simulink model "uz_ParameterID6ph"  (R2021b)
settings: Solver=FixedStepDiscrete  StartTime=0.0  StopTime=160  FixedStep=0.000005  RelTol=1e-3  EnableMultiTasking=on
model workspace (MATLAB code in the model file):
  | cmdLim = Simulink.Parameter;
  | cmdLim.Value = 15;
  | cmdLim.Description = 'Limit for controlling the maximum surface command angle.';
  | cmdLim.Min = 0;
  | cmdLim.Max = 90;
  | cmdLim.DocUnits = 'deg';
  | 
  | dispGain = Simulink.Parameter;
  | dispGain.Value = 0.75;
  | dispGain.Description = 'Gain applied to the displacement error.';
  | dispGain.Min = 0;
  | dispGain.Max = [];
  | dispGain.DocUnits = 'deg/sec/deg';
  | 
  | dispLim = Simulink.Parameter;
  | dispLim.Value = 30;
  | dispLim.Description = 'Limit for controlling the maximum commanded angle.';
  | dispLim.Min = 0;
  | dispLim.Max = 180;
  | dispLim.DocUnits = 'deg';
  | 
  | intGain = Simulink.Parameter;
  | intGain.Value = 0.5;
  | intGain.Description = 'Gain applied to the integral error.';
  | intGain.Min = 0;
  | intGain.Max = [];
  | intGain.DocUnits = 'deg/sec/deg/sec';
  | 
  | intLim = Simulink.Parameter;
  | intLim.Value = 5;
  | intLim.Description = 'Limit for controlling the maximum commanded angle.';
  | intLim.Min = 0;
  | intLim.Max = 90;
  | intLim.DocUnits = 'deg';
  | 
  | rateGain = Simulink.Parameter;
  | rateGain.Value = 2;
  | rateGain.Description = 'Gain applied to the rate error.';
  | rateGain.Min = 0;
  | rateGain.Max = [];
  | rateGain.DocUnits = 'deg/deg/sec';
  | 
  | rateLim = Simulink.Parameter;
  | rateLim.Value = 6;
  | rateLim.Description = 'Limit for controlling the maximum commanded angle.';
  | rateLim.Min = 0;
  | rateLim.Max = 180;
  | rateLim.DocUnits = 'deg/sec';
  | 
  | hdgGain = Simulink.Parameter;
  | hdgGain.Value = 0.015;
values from neighbouring files (symbols this model uses):
  c = 2/6*cat(1,tl1,tl2,tl3,tl4,tl5,tl6)    [Parameter_Init_Buehler_201_6ph.m]
  d_d_TMS = 0.005    [Parameter_Init_Buehler_201.m]
  d_f_hardware = 200000    [Parameter_Init_Buehler_201.m]
  d_f_states = 20000    [Parameter_Init_Buehler_201.m]
  d_i_max = 15    [Parameter_Init_Buehler_201.m]
  d_i_min = -d_i_max    (= -15)    [Parameter_Init_Buehler_201.m]
  d_I_n = 8    [Parameter_Init_Buehler_201.m]
  d_J_Coupling_M_E = 2e-6    (= 2e-06)    [Parameter_Init_Buehler_201.m]
  d_J_Coupling_M_Ms = 2e-20    [Parameter_Init_Buehler_201.m]
  d_J_Ms_L = d_J_Ms_M    (= 1.26363648e-05)    [Parameter_Init_Buehler_201.m]
  d_J_Ms_M = 0.5*0.5*((0.5*d_d_Ms)^4)*3.14*d_l_Ms*d_rho_Ms    (= 1.26363648e-05)    [Parameter_Init_Buehler_201.m]
  d_Ki_id = 162.47    [Parameter_Init_Buehler_201.m]
  d_Ki_iq = 162.47    [Parameter_Init_Buehler_201.m]
  d_Ki_n = 1.982    [Parameter_Init_Buehler_201.m]
  d_Kp_id = 0.369    [Parameter_Init_Buehler_201.m]
  d_Kp_iq = 0.369    [Parameter_Init_Buehler_201.m]
  d_Kp_n = 0.198    [Parameter_Init_Buehler_201.m]
  d_L_d = 0.00031    [Parameter_Init_Buehler_201.m]
  d_L_q = 0.00033    [Parameter_Init_Buehler_201.m]
  d_n_n = 3200    [Parameter_Init_Buehler_201.m]
  d_p = 4    [Parameter_Init_Buehler_201.m]
  d_psi_pm = 0.0075    [Parameter_Init_Buehler_201.m]
  d_R_ph = d_R_ph_ph/2    (= 0.089)    [Parameter_Init_Buehler_201.m]
  d_y_max = 10    [Parameter_Init_Buehler_201.m]
  d_y_min = -d_y_max    (= -10)    [Parameter_Init_Buehler_201.m]
  V_DC = 24    [Parameter_Init_Buehler_201.m]
undefined symbols (not defined in the file or in its folder): i_dq, i_dq_ref, n_ref, ts_ps, V_abc, v_dq
libraries: fl_lib x66, nesl_utility x51, ee_lib x38, simulink x14, spsTriangleGeneratorLib x3, spsabctodq0Lib x2, spsAlphaBetaZerotodq0Lib x2, spsdq0toabcLib x1
(part 5 of 6)

== system uz_ParameterID6ph/Hardware/coupling m. shaft/Inertia ==
  Trägheitsmoment3 : fl_lib/Mechanical/Rotational Elements/Inertia  Commented=on  inertia=d_J_Coupling_M_Ms kg*m^2  num_ports=foundation.enum.numPorts2.one  w_specify=off  w_priority=High  w=0 rad/s  w_nominal_specify=off  w_nominal_unit=rad/s  w_nominal_value=1  t_specify=off  t_priority=None  t=0 N*m  t_nominal_specify=off  t_nominal_unit=N*m  t_nominal_value=1
      settings: AttributesFormatString=J in [%<inertia_unit>]
  Input : PMIOPort  Side=Left
  output : PMIOPort  Port=2  Side=Right
  connections:
  Input/RConn1 -- Trägheitsmoment3/LConn1 -- output/RConn1

== system uz_ParameterID6ph/Hardware/coupling m. shaft/Spring Damper System ==
  Rotational Spring : fl_lib/Mechanical/Rotational Elements/Rotational Spring  spr_rate=d_c_Coupling_M_Ms N*m/rad  w_specify=off  w_priority=None  w=0 rad/s  w_nominal_specify=off  w_nominal_unit=rad/s  w_nominal_value=1  t_specify=off  t_priority=None  t=0 N*m  t_nominal_specify=off  t_nominal_unit=N*m  t_nominal_value=1  phi_specify=off  phi_priority=High  phi=0 rad  phi_nominal_specify=off  phi_nominal_unit=rad  phi_nominal_value=1
  Trägheitsmoment1 : fl_lib/Mechanical/Rotational Elements/Inertia  inertia=d_J_Coupling_M_Ms/2 kg*m^2  num_ports=foundation.enum.numPorts2.one  w_specify=off  w_priority=High  w=0 rad/s  w_nominal_specify=off  w_nominal_unit=rad/s  w_nominal_value=1  t_specify=off  t_priority=None  t=0 N*m  t_nominal_specify=off  t_nominal_unit=N*m  t_nominal_value=1
      settings: AttributesFormatString=J in [%<inertia_unit>]
  Trägheitsmoment3 : fl_lib/Mechanical/Rotational Elements/Inertia  inertia=d_J_Coupling_M_Ms/2 kg*m^2  num_ports=foundation.enum.numPorts2.one  w_specify=off  w_priority=High  w=0 rad/s  w_nominal_specify=off  w_nominal_unit=rad/s  w_nominal_value=1  t_specify=off  t_priority=None  t=0 N*m  t_nominal_specify=off  t_nominal_unit=N*m  t_nominal_value=1
      settings: AttributesFormatString=J in [%<inertia_unit>]
  dm : fl_lib/Mechanical/Rotational Elements/Rotational Damper  Commented=on  D=0 N*m/(rad/s)  w_specify=off  w_priority=None  w=0 rad/s  w_nominal_specify=off  w_nominal_unit=rad/s  w_nominal_value=1  t_specify=off  t_priority=None  t=0 N*m  t_nominal_specify=off  t_nominal_unit=N*m  t_nominal_value=1
  Input : PMIOPort  Side=Left
  output : PMIOPort  Port=2  Side=Right
  connections:
  Rotational Spring/LConn1 -- dm/LConn1 -- Input/RConn1 -- Trägheitsmoment3/LConn1
  Trägheitsmoment1/LConn1 -- Rotational Spring/RConn1 -- dm/RConn1 -- output/RConn1

== system uz_ParameterID6ph/Hardware1/maschine_models/Connected_VSD ==
  Mechanical Rotational Reference2 : fl_lib/Mechanical/Rotational Elements/Mechanical Rotational Reference
  Open Circuit : fl_lib/Electrical/Electrical Elements/Open Circuit  v_specify=off  v_priority=None  v=0 V  v_nominal_specify=off  v_nominal_unit=V  v_nominal_value=1
      settings: SourceProductBaseCode=SS
  Phase Splitter3 : ee_lib/Connectors & References/Phase Splitter
      settings: SourceProductBaseCode=PS
  Phase Splitter4 : ee_lib/Connectors & References/Phase Splitter
      settings: SourceProductBaseCode=PS
  Simscape Component1 : SimscapeComponentBlock  SourceFile=PMSM_6ph_VSD_Rockhill_singleN  ComponentPath=PMSM_6ph_VSD_Rockhill_singleN  ComponentVariants="[\"PMSM_6ph_VSD_Rockhill_singleN\"]"  ComponentVariantNames="[\"PMSM_6ph_VSD_Rockhill_singleN\"]"  ClassName=PMSM_6ph_VSD_Rockhill_singleN  SchemaVersion=1  psi_pm=1 Wb  L_d=1 H  L_q=1 H  L_ls=0.00016 H  Rs=1 Ohm  p=1  n=9  i_a1_specify=off  i_a1_priority=None  i_a1=0 A  i_a1_nominal_specify=off  i_a1_nominal_unit=A  i_a1_nominal_value=1  i_b1_specify=off  i_b1_priority=None  i_b1=0 A  i_b1_nominal_specify=off  i_b1_nominal_unit=A  i_b1_nominal_value=1  i_c1_specify=off  i_c1_priority=None  i_c1=0 A  i_c1_nominal_specify=off  i_c1_nominal_unit=A  i_c1_nominal_value=1  i_a2_specify=off  i_a2_priority=None  i_a2=0 A  i_a2_nominal_specify=off  i_a2_nominal_unit=A  i_a2_nominal_value=1  i_b2_specify=off  i_b2_priority=None  i_b2=0 A  i_b2_nominal_specify=off  i_b2_nominal_unit=A  i_b2_nominal_value=1  i_c2_specify=off  i_c2_priority=None  i_c2=0 A  i_c2_nominal_specify=off  i_c2_nominal_unit=A  i_c2_nominal_value=1  i_d_specify=off  i_d_priority=None  i_d=0 A  i_d_nominal_specify=off  i_d_nominal_unit=A  i_d_nominal_value=1  i_q_specify=off  i_q_priority=None  i_q=0 A  i_q_nominal_specify=off  i_q_nominal_unit=A  i_q_nominal_value=1  i_a_specify=off  i_a_priority=None  i_a=0 A  i_a_nominal_specify=off  i_a_nominal_unit=A  i_a_nominal_value=1  i_b_specify=off  i_b_priority=None  i_b=0 A  i_b_nominal_specify=off  i_b_nominal_unit=A  i_b_nominal_value=1  i_x_specify=off  i_x_priority=None  i_x=0 A  i_x_nominal_specify=off  i_x_nominal_unit=A  i_x_nominal_value=1  i_y_specify=off  i_y_priority=None  i_y=0 A  i_y_nominal_specify=off  i_y_nominal_unit=A  i_y_nominal_value=1  i_zp_specify=off  i_zp_priority=None  i_zp=0 A  i_zp_nominal_specify=off  i_zp_nominal_unit=A  i_zp_nominal_value=1  i_zm_specify=off  i_zm_priority=None  i_zm=0 A  i_zm_nominal_specify=off  i_zm_nominal_unit=A  i_zm_nominal_value=1  u_d_specify=off  u_d_priority=None  u_d=0 V  u_d_nominal_specify=off  u_d_nominal_unit=V  u_d_nominal_value=1  u_q_specify=off  u_q_priority=None  u_q=0 V  u_q_nominal_specify=off  u_q_nominal_unit=V  u_q_nominal_value=1  u_a_specify=off  u_a_priority=None  u_a=0 V  u_a_nominal_specify=off  u_a_nominal_unit=V  u_a_nominal_value=1  u_b_specify=off  u_b_priority=None  u_b=0 V  u_b_nominal_specify=off  u_b_nominal_unit=V  u_b_nominal_value=1  u_x_specify=off  u_x_priority=None  u_x=0 V  u_x_nominal_specify=off  u_x_nominal_unit=V  u_x_nominal_value=1  u_y_specify=off  u_y_priority=None  u_y=0 V  u_y_nominal_specify=off  u_y_nominal_unit=V  u_y_nominal_value=1  u_zp_specify=off  u_zp_priority=None  u_zp=0 V  u_zp_nominal_specify=off  u_zp_nominal_unit=V  u_zp_nominal_value=1  u_zm_specify=off  u_zm_priority=None  u_zm=0 V  u_zm_nominal_specify=off  u_zm_nominal_unit=V  u_zm_nominal_value=1  m_m_specify=off  m_m_priority=None  m_m=0 N*m  m_m_nominal_specify=off  m_m_nominal_unit=N*m  m_m_nominal_value=1  theta_specify=off  theta_priority=None  theta=0 rad  theta_nominal_specify=off  theta_nominal_unit=rad  theta_nominal_value=1
      settings: CopyFcn=simscape.engine.sli.internal.componentblockcallback(gcbh,'COPY')  PreCopyFcn=simscape.engine.sli.internal.componentblockcallback(gcbh,'PRECOPY')  PreDeleteFcn=simscape.engine.sli.internal.componentblockcallback(gcbh,'PREDELETE')  InternalSimscapePortConfiguration="{\"Bottom\":[],\"Left\":[{\"id\":\"a1\",\"label\":\"a1\",\"type\":\"foundation.electrical.electrical\"},{\"id\":\"b1\",\"label\":\"b1\",\"type\":\"foundation.electrical.electrical\"},{\"id\":\"c1\",\"label\":\"c1\",\"type\":\"foundation.electrical.electrical\"},{\"id\":\"a2\",\"label\":\"a2\",\"type\":\"foundation.electrical.electrical\"},{\"id\":\"b2\",\"label\":\"b2\",\"type\":\"foundation.electrical.electrical\"},{\"id\":\"c2\",\"label\":\"c2\",\"type\":\"foundation.electrical.electrical\"},{\"id\":\"neutral\",\"label\":\"neutral\",\"type\":\"foundation.electrical.electrical\"}],\"Right\":[{\"id\":\"Rot\",\"label\":\"Rot\",\"type\":\"foundation.mechanical.rotational.rotational\"},{\"id\":\"Case\",\"label\":\"Case\",\"type\":\"foundation.mechanical.rotational.rotational\"}],\"Top\":[]}"
      mask Type: PMSM_6ph_VSD_Rockhill_singleN
  System1 : PMIOPort  Side=Left
  Rot : PMIOPort  Port=2  Side=Right
  System2 : PMIOPort  Port=3  Side=Left
  connections:
  Open Circuit/LConn1 -- Simscape Component1/LConn7
  Simscape Component1/LConn6 -- Phase Splitter4/RConn3
  Phase Splitter3/RConn2 -- Simscape Component1/LConn2
  Phase Splitter3/RConn1 -- Simscape Component1/LConn1
  Phase Splitter3/RConn3 -- Simscape Component1/LConn3
  Simscape Component1/LConn4 -- Phase Splitter4/RConn1
  Simscape Component1/LConn5 -- Phase Splitter4/RConn2
  Mechanical Rotational Reference2/LConn1 -- Simscape Component1/RConn2
  Phase Splitter4/LConn1 -- System2/RConn1
  Phase Splitter3/LConn1 -- System1/RConn1
  Simscape Component1/RConn1 -- Rot/RConn1

== system uz_ParameterID6ph/Hardware1/maschine_models/Isolated_VSD ==
  Mechanical Rotational Reference1 : fl_lib/Mechanical/Rotational Elements/Mechanical Rotational Reference
  Open Circuit : fl_lib/Electrical/Electrical Elements/Open Circuit  v_specify=off  v_priority=None  v=0 V  v_nominal_specify=off  v_nominal_unit=V  v_nominal_value=1
      settings: SourceProductBaseCode=SS
  Open Circuit1 : fl_lib/Electrical/Electrical Elements/Open Circuit  v_specify=off  v_priority=None  v=0 V  v_nominal_specify=off  v_nominal_unit=V  v_nominal_value=1
      settings: SourceProductBaseCode=SS
  Phase Splitter : ee_lib/Connectors & References/Phase Splitter
      settings: SourceProductBaseCode=PS
  Phase Splitter1 : ee_lib/Connectors & References/Phase Splitter
      settings: SourceProductBaseCode=PS
  Simscape Component : SimscapeComponentBlock  SourceFile=PMSM_6ph_VSD_Rockhill_isolatedN  ComponentPath=PMSM_6ph_VSD_Rockhill_isolatedN  ComponentVariants="[\"PMSM_6ph_VSD_Rockhill_isolatedN\"]"  ComponentVariantNames="[\"PMSM_6ph_VSD_Rockhill_isolatedN\"]"  ClassName=PMSM_6ph_VSD_Rockhill_isolatedN  SchemaVersion=1  psi_pm=d_psi_pm Wb  L_d=d_L_d H  L_q=d_L_q H  L_ls=d_L_0 H  Rs=d_R_ph Ohm  p=d_p  n=6  theta_offset=0.5 rad  i_a1_specify=off  i_a1_priority=None  i_a1=0 A  i_a1_nominal_specify=off  i_a1_nominal_unit=A  i_a1_nominal_value=1  i_b1_specify=off  i_b1_priority=None  i_b1=0 A  i_b1_nominal_specify=off  i_b1_nominal_unit=A  i_b1_nominal_value=1  i_c1_specify=off  i_c1_priority=None  i_c1=0 A  i_c1_nominal_specify=off  i_c1_nominal_unit=A  i_c1_nominal_value=1  i_a2_specify=off  i_a2_priority=None  i_a2=0 A  i_a2_nominal_specify=off  i_a2_nominal_unit=A  i_a2_nominal_value=1  i_b2_specify=off  i_b2_priority=None  i_b2=0 A  i_b2_nominal_specify=off  i_b2_nominal_unit=A  i_b2_nominal_value=1  i_c2_specify=off  i_c2_priority=None  i_c2=0 A  i_c2_nominal_specify=off  i_c2_nominal_unit=A  i_c2_nominal_value=1  i_d_specify=off  i_d_priority=None  i_d=0 A  i_d_nominal_specify=off  i_d_nominal_unit=A  i_d_nominal_value=1  i_q_specify=off  i_q_priority=None  i_q=0 A  i_q_nominal_specify=off  i_q_nominal_unit=A  i_q_nominal_value=1  i_a_specify=off  i_a_priority=None  i_a=0 A  i_a_nominal_specify=off  i_a_nominal_unit=A  i_a_nominal_value=1  i_b_specify=off  i_b_priority=None  i_b=0 A  i_b_nominal_specify=off  i_b_nominal_unit=A  i_b_nominal_value=1  i_x_specify=off  i_x_priority=None  i_x=0 A  i_x_nominal_specify=off  i_x_nominal_unit=A  i_x_nominal_value=1  i_y_specify=off  i_y_priority=None  i_y=0 A  i_y_nominal_specify=off  i_y_nominal_unit=A  i_y_nominal_value=1  i_zp_specify=off  i_zp_priority=None  i_zp=0 A  i_zp_nominal_specify=off  i_zp_nominal_unit=A  i_zp_nominal_value=1  i_zm_specify=off  i_zm_priority=None  i_zm=0 A  i_zm_nominal_specify=off  i_zm_nominal_unit=A  i_zm_nominal_value=1  u_d_specify=off  u_d_priority=None  u_d=0 V  u_d_nominal_specify=off  u_d_nominal_unit=V  u_d_nominal_value=1  u_q_specify=off  u_q_priority=None  u_q=0 V  u_q_nominal_specify=off  u_q_nominal_unit=V  u_q_nominal_value=1  u_a_specify=off  u_a_priority=None  u_a=0 V  u_a_nominal_specify=off  u_a_nominal_unit=V  u_a_nominal_value=1  u_b_specify=off  u_b_priority=None  u_b=0 V  u_b_nominal_specify=off  u_b_nominal_unit=V  u_b_nominal_value=1  u_x_specify=off  u_x_priority=None  u_x=0 V  u_x_nominal_specify=off  u_x_nominal_unit=V  u_x_nominal_value=1  u_y_specify=off  u_y_priority=None  u_y=0 V  u_y_nominal_specify=off  u_y_nominal_unit=V  u_y_nominal_value=1  u_zp_specify=off  u_zp_priority=None  u_zp=0 V  u_zp_nominal_specify=off  u_zp_nominal_unit=V  u_zp_nominal_value=1  u_zm_specify=off  u_zm_priority=None  u_zm=0 V  u_zm_nominal_specify=off  u_zm_nominal_unit=V  u_zm_nominal_value=1  m_m_specify=off  m_m_priority=None  m_m=0 N*m  m_m_nominal_specify=off  m_m_nominal_unit=N*m  m_m_nominal_value=1  theta_specify=off  theta_priority=None  theta=0 rad  theta_nominal_specify=off  theta_nominal_unit=rad  theta_nominal_value=1
      settings: CopyFcn=simscape.engine.sli.internal.componentblockcallback(gcbh,'COPY')  PreCopyFcn=simscape.engine.sli.internal.componentblockcallback(gcbh,'PRECOPY')  PreDeleteFcn=simscape.engine.sli.internal.componentblockcallback(gcbh,'PREDELETE')  InternalSimscapePortConfiguration="{\"Bottom\":[],\"Left\":[{\"id\":\"a1\",\"label\":\"a1\",\"type\":\"foundation.electrical.electrical\"},{\"id\":\"b1\",\"label\":\"b1\",\"type\":\"foundation.electrical.electrical\"},{\"id\":\"c1\",\"label\":\"c1\",\"type\":\"foundation.electrical.electrical\"},{\"id\":\"n1\",\"label\":\"n1\",\"type\":\"foundation.electrical.electrical\"},{\"id\":\"a2\",\"label\":\"a2\",\"type\":\"foundation.electrical.electrical\"},{\"id\":\"b2\",\"label\":\"b2\",\"type\":\"foundation.electrical.electrical\"},{\"id\":\"c2\",\"label\":\"c2\",\"type\":\"foundation.electrical.electrical\"},{\"id\":\"n2\",\"label\":\"n2\",\"type\":\"foundation.electrical.electrical\"}],\"Right\":[{\"id\":\"Rot\",\"label\":\"Rot\",\"type\":\"foundation.mechanical.rotational.rotational\"},{\"id\":\"Case\",\"label\":\"Case\",\"type\":\"foundation.mechanical.rotational.rotational\"}],\"Top\":[]}"
      mask Type: PMSM_6ph_VSD_Rockhill_isolatedN
  System1 : PMIOPort  Side=Left
  Rot : PMIOPort  Port=2  Side=Right
  System2 : PMIOPort  Port=3  Side=Left
  connections:
  Phase Splitter/LConn1 -- System1/RConn1
  Phase Splitter1/RConn1 -- Simscape Component/LConn5
  Phase Splitter/RConn3 -- Simscape Component/LConn3
  Phase Splitter1/RConn2 -- Simscape Component/LConn6
  Phase Splitter1/RConn3 -- Simscape Component/LConn7
  Phase Splitter/RConn2 -- Simscape Component/LConn2
  Simscape Component/RConn1 -- Rot/RConn1
  Simscape Component/LConn1 -- Phase Splitter/RConn1
  System2/RConn1 -- Phase Splitter1/LConn1
  Mechanical Rotational Reference1/LConn1 -- Simscape Component/RConn2
  Open Circuit/LConn1 -- Simscape Component/LConn4
  Open Circuit1/LConn1 -- Simscape Component/LConn8

== system uz_ParameterID6ph/Hardware1/setpoint/rpm_setpoint ==
  setpoint : Inport
  Gain8 : Gain  Gain=pi/30  OutDataTypeStr=double
  Ideal Angular Velocity Source1 : fl_lib/Mechanical/Mechanical Sources/Ideal Angular Velocity Source
  Mechanical Rotational Reference5 : fl_lib/Mechanical/Rotational Elements/Mechanical Rotational Reference
  Simulink-PS Converter10 : nesl_utility/Simulink-PS Converter  PhysicalDomain=network_engine_domain  SubClassName=ps_input  LeftPortType=input  RightPortType=output  PseudoPeriodic=off  Frequencies=[]  NoiseDistribution=none  NoiseParameters=[]  Unit=1  AffineConversion=off  FilteringAndDerivatives=filter  SimscapeFilterOrder=1  InputFilterTimeConstant=0.001  UdotUserProvided=0
      settings: SourceProductBaseCode=PW,SS
  rpm : PMIOPort  Side=Right
  wires:
  setpoint/1 -> Gain8/1
  Gain8/1 -> Simulink-PS Converter10/1
  connections:
  rpm/RConn1 -- Ideal Angular Velocity Source1/LConn1
  Simulink-PS Converter10/RConn1 -- Ideal Angular Velocity Source1/RConn1
  Mechanical Rotational Reference5/LConn1 -- Ideal Angular Velocity Source1/RConn2

== system uz_ParameterID6ph/Hardware1/setpoint/torque_load ==
  setpoint : Inport
  Ideal Torque Source : fl_lib/Mechanical/Mechanical Sources/Ideal Torque Source
  Mechanical Rotational Reference6 : fl_lib/Mechanical/Rotational Elements/Mechanical Rotational Reference
  S1 : nesl_utility/Simulink-PS Converter  PhysicalDomain=network_engine_domain  SubClassName=ps_input  LeftPortType=input  RightPortType=output  PseudoPeriodic=off  Frequencies=[]  NoiseDistribution=none  NoiseParameters=[]  Unit=1  AffineConversion=off  FilteringAndDerivatives=provide  SimscapeFilterOrder=1  InputFilterTimeConstant=0.001  UdotUserProvided=0
      settings: SourceProductBaseCode=PW,SS
  torque : PMIOPort  Side=Right
  wires:
  setpoint/1 -> S1/1
  connections:
  S1/RConn1 -- Ideal Torque Source/RConn1
  torque/RConn1 -- Ideal Torque Source/LConn1
  Mechanical Rotational Reference6/LConn1 -- Ideal Torque Source/RConn2

== system uz_ParameterID6ph/FOC/uz_FOC_Current/id-PI-Controller with anti wind-up/Clamping circuit ==
  preSat : Inport  DisableCoverage=on  OutDataTypeStr=single
  preIntegrator : Inport  DisableCoverage=on  Port=2
  AND : Logic  DisableCoverage=on
  DataTypeConv1 : DataTypeConversion  DisableCoverage=on  OutDataTypeStr=int8  SaturateOnIntegerOverflow=on  RndMeth=Zero  LockScale=on
  DataTypeConv2 : DataTypeConversion  DisableCoverage=on  OutDataTypeStr=int8  SaturateOnIntegerOverflow=on  RndMeth=Zero  LockScale=on
  DeadZone : DeadZone  DisableCoverage=on  LowerValue=d_y_min  UpperValue=d_y_max  SaturateOnIntegerOverflow=on
  Equal : RelationalOperator  DisableCoverage=on  Operator===  RndMeth=Nearest  InputSameDT=on
  NotEqual : RelationalOperator  DisableCoverage=on  Operator=~=  RndMeth=Nearest  InputSameDT=on
  SignDeltaU : Signum  DisableCoverage=on
  SignPreIntegrator : Signum  DisableCoverage=on
  ZeroGain : Gain  DisableCoverage=on  Gain=0  ParamDataTypeStr=double  OutDataTypeStr=single  SaturateOnIntegerOverflow=on
  Clamp : Outport  DisableCoverage=on  VectorParamsAs1DForOutWhenUnconnected=off
  wires:
  preSat/1 -> ZeroGain/1, DeadZone/1
  preIntegrator/1 -> SignPreIntegrator/1
  ZeroGain/1 -> NotEqual/1
  DeadZone/1 -> NotEqual/2, SignDeltaU/1
  SignDeltaU/1 -> DataTypeConv1/1
  DataTypeConv1/1 -> Equal/1
  SignPreIntegrator/1 -> DataTypeConv2/1
  DataTypeConv2/1 -> Equal/2
  NotEqual/1 -> AND/1
  Equal/1 -> AND/2
  AND/1 -> Clamp/1

== system uz_ParameterID6ph/FOC/uz_FOC_Current/iq-PI-Controller with anti wind-up/Clamping circuit ==
  preSat : Inport  DisableCoverage=on  OutDataTypeStr=single
  preIntegrator : Inport  DisableCoverage=on  Port=2
  AND : Logic  DisableCoverage=on
  DataTypeConv1 : DataTypeConversion  DisableCoverage=on  OutDataTypeStr=int8  SaturateOnIntegerOverflow=on  RndMeth=Zero  LockScale=on
  DataTypeConv2 : DataTypeConversion  DisableCoverage=on  OutDataTypeStr=int8  SaturateOnIntegerOverflow=on  RndMeth=Zero  LockScale=on
  DeadZone : DeadZone  DisableCoverage=on  LowerValue=d_y_min  UpperValue=d_y_max  SaturateOnIntegerOverflow=on
  Equal : RelationalOperator  DisableCoverage=on  Operator===  RndMeth=Nearest  InputSameDT=on
  NotEqual : RelationalOperator  DisableCoverage=on  Operator=~=  RndMeth=Nearest  InputSameDT=on
  SignDeltaU : Signum  DisableCoverage=on
  SignPreIntegrator : Signum  DisableCoverage=on
  ZeroGain : Gain  DisableCoverage=on  Gain=0  ParamDataTypeStr=double  OutDataTypeStr=single  SaturateOnIntegerOverflow=on
  Clamp : Outport  DisableCoverage=on  VectorParamsAs1DForOutWhenUnconnected=off
  wires:
  preSat/1 -> ZeroGain/1, DeadZone/1
  preIntegrator/1 -> SignPreIntegrator/1
  ZeroGain/1 -> NotEqual/1
  DeadZone/1 -> NotEqual/2, SignDeltaU/1
  SignDeltaU/1 -> DataTypeConv1/1
  DataTypeConv1/1 -> Equal/1
  SignPreIntegrator/1 -> DataTypeConv2/1
  DataTypeConv2/1 -> Equal/2
  NotEqual/1 -> AND/1
  Equal/1 -> AND/2
  AND/1 -> Clamp/1

== system uz_ParameterID6ph/FOC/uz_FOC_Speed/omega-PI-Controller with anti wind-up/Clamping circuit ==
  preSat : Inport  DisableCoverage=on  OutDataTypeStr=single
  preIntegrator : Inport  DisableCoverage=on  Port=2
  AND : Logic  DisableCoverage=on
  DataTypeConv1 : DataTypeConversion  DisableCoverage=on  OutDataTypeStr=int8  SaturateOnIntegerOverflow=on  RndMeth=Zero  LockScale=on
  DataTypeConv2 : DataTypeConversion  DisableCoverage=on  OutDataTypeStr=int8  SaturateOnIntegerOverflow=on  RndMeth=Zero  LockScale=on
  DeadZone : DeadZone  DisableCoverage=on  LowerValue=d_i_min  UpperValue=d_i_max  SaturateOnIntegerOverflow=on
  Equal : RelationalOperator  DisableCoverage=on  Operator===  RndMeth=Nearest  InputSameDT=on
  NotEqual : RelationalOperator  DisableCoverage=on  Operator=~=  RndMeth=Nearest  InputSameDT=on
  SignDeltaU : Signum  DisableCoverage=on
  SignPreIntegrator : Signum  DisableCoverage=on
  ZeroGain : Gain  DisableCoverage=on  Gain=0  ParamDataTypeStr=double  OutDataTypeStr=single  SaturateOnIntegerOverflow=on
  Clamp : Outport  DisableCoverage=on  VectorParamsAs1DForOutWhenUnconnected=off
  wires:
  preSat/1 -> ZeroGain/1, DeadZone/1
  preIntegrator/1 -> SignPreIntegrator/1
  ZeroGain/1 -> NotEqual/1
  DeadZone/1 -> NotEqual/2, SignDeltaU/1
  SignDeltaU/1 -> DataTypeConv1/1
  DataTypeConv1/1 -> Equal/1
  SignPreIntegrator/1 -> DataTypeConv2/1
  DataTypeConv2/1 -> Equal/2
  NotEqual/1 -> AND/1
  Equal/1 -> AND/2
  AND/1 -> Clamp/1

== matlab function uz_ParameterID6ph/Hardware/12bit ADC1 ==
  data: u input; y output
function y = fcn(u)
%#codegen

y = u*2048/5;

== matlab function uz_ParameterID6ph/Hardware/12bit ADC ==
  data: u input; y output
function y = fcn(u)
%#codegen

y = u*2048/5;

== matlab function uz_ParameterID6ph/Hardware/12bit ADC2 ==
  data: u input; y output
function y = fcn(u)
%#codegen

y = u*2048/5;

== matlab function uz_ParameterID6ph/FOC/Busselector ==
  data: ControlFlags input Bus: uz_ParaID_ControlFlags_t; FOC_state_outputs output Bus: uz_ParaID_Controller_Parameters_output_t; ElectricalID_FOC_input input Bus: uz_ParaID_Controller_Parameters_output_t; FrictionID_FOC_input input Bus: uz_ParaID_Controller_Parameters_output_t; FluxMapID_FOC_input input Bus: uz_ParaID_Controller_Parameters_output_t; TwoMassID_FOC_input input Bus: uz_ParaID_Controller_Parameters_output_t; FOCControl_input input Bus: uz_ParaID_Controller_Parameters_output_t
function FOC_state_outputs = fcn(ControlFlags,ElectricalID_FOC_input,....
    FrictionID_FOC_input,FluxMapID_FOC_input,TwoMassID_FOC_input,FOCControl_input)

switch ControlFlags.transNr
    case 0
        if(ControlFlags.finished_all_Offline_states==1)
            FOC_state_outputs           = FOCControl_input;
        else
        FOC_state_outputs.i_dq_ref.d          = single(0);
        FOC_state_outputs.i_dq_ref.q          = single(0);
        FOC_state_outputs.i_dq_ref.zero       = single(0);
        FOC_state_outputs.activeState         = uint16(0);
        FOC_state_outputs.n_ref_FOC           = single(0);
        FOC_state_outputs.enableFOC_speed     = boolean(0);
        FOC_state_outputs.enableFOC_current   = boolean(0);
        FOC_state_outputs.resetIntegrator     = boolean(0);
        FOC_state_outputs.Kp_id_out           = single(0);
        FOC_state_outputs.Kp_iq_out           = single(0);
        FOC_state_outputs.Kp_n_out            = single(0);
        FOC_state_outputs.Ki_id_out           = single(0);
        FOC_state_outputs.Ki_iq_out           = single(0);
        FOC_state_outputs.Ki_n_out            = single(0);
        end
    case 1
        FOC_state_outputs           = ElectricalID_FOC_input;
    case 2
        FOC_state_outputs           = TwoMassID_FOC_input;
    case 3
        FOC_state_outputs           = FrictionID_FOC_input;
    case 4
        FOC_state_outputs           = FluxMapID_FOC_input;
    otherwise
        FOC_state_outputs.i_dq_ref.d          = single(0);
        FOC_state_outputs.i_dq_ref.q          = single(0);
        FOC_state_outputs.i_dq_ref.zero       = single(0);
        FOC_state_outputs.activeState         = uint16(0);
        FOC_state_outputs.n_ref_FOC           = single(0);
        FOC_state_outputs.enableFOC_speed     = boolean(0);
        FOC_state_outputs.enableFOC_current   = boolean(0);
        FOC_state_outputs.resetIntegrator     = boolean(0);
        FOC_state_outputs.Kp_id_out           = single(0);
        FOC_state_outputs.Kp_iq_out           = single(0);
        FOC_state_outputs.Kp_n_out            = single(0);
        FOC_state_outputs.Ki_id_out           = single(0);
        FOC_state_outputs.Ki_iq_out           = single(0);
        FOC_state_outputs.Ki_n_out            = single(0);
end
end

== stateflow chart uz_ParameterID6ph/ControlState ==
  settings: updateMethod=DISCRETE  sampleTime=1/d_f_states
  note: ControlState
  state ControlState
    entry:
    during:
    GlobalConfig_out.Reset = GlobalConfig_in.Reset;
    GlobalConfig_out.ACCEPT = GlobalConfig_in.ACCEPT;
    GlobalConfig_out.enableParameterID = GlobalConfig_in.enableParameterID;
    GlobalConfig_out.ElectricalID = GlobalConfig_in.ElectricalID;
    GlobalConfig_out.FrictionID = GlobalConfig_in.FrictionID
    GlobalConfig_out.TwoMassID = GlobalConfig_in.TwoMassID;
    GlobalConfig_out.FluxMapID = GlobalConfig_in.FluxMapID;
    GlobalConfig_out.OnlineID = GlobalConfig_in.OnlineID;
    GlobalConfig_out.sampleTimeISR = GlobalConfig_in.sampleTimeISR;
    state decideMotorID
      entry:
      during:
      if (GlobalConfig_in.ACCEPT == 1)
      decideIDstates;
      end
      if(ControlFlags.finished_all_Offline_states == 1 && GlobalConfig_in.OnlineID==1 && enteredOnlineID==0)
      ControlFlags.enableOnlineID=boolean(1);
      elseif (ControlFlags.finished_all_Offline_states == 1 && GlobalConfig_in.OnlineID==0 && enteredOnlineID==1)
      ControlFlags.enableOnlineID=boolean(0);
      end
      exit:
    state activateFrictionID
      entry:
      ControlFlags.startFrictionID=boolean(1);
      during:
      exit:
    state activateFluxMapID
      entry:
      ControlFlags.startFluxMapID=boolean(1);
      during:
      exit:
    state activateTwoMassID
      entry:
      ControlFlags.startTwoMassID=boolean(1);
      during:
      exit:
    state activateElectricalID
      entry:
      ControlFlags.startElectricalID=boolean(1);
      during:
      exit:
    state duringElectricalID
      entry:
      ControlFlags.startElectricalID=boolean(0);
      during:
      GlobalConfig_out.PMSM_config.Ld_Henry=ElectricalID_output.PMSM_parameters.Ld_Henry;
      GlobalConfig_out.PMSM_config.Lq_Henry=ElectricalID_output.PMSM_parameters.Lq_Henry;
      GlobalConfig_out.PMSM_config.R_ph_Ohm=ElectricalID_output.PMSM_parameters.R_ph_Ohm;
      GlobalConfig_out.PMSM_config.Psi_PM_Vs=ElectricalID_output.PMSM_parameters.Psi_PM_Vs;
      GlobalConfig_out.PMSM_config.polePairs=ElectricalID_output.PMSM_parameters.polePairs;
      GlobalConfig_out.PMSM_config.J_kg_m_squared=....
      ElectricalID_output.PMSM_parameters.J_kg_m_squared;
      GlobalConfig_out.Kp_id=ElectricalID_FOC_output.Kp_id_out;
      GlobalConfig_out.Kp_iq=ElectricalID_FOC_output.Kp_iq_out;
      GlobalConfig_out.Kp_n=ElectricalID_FOC_output.Kp_n_out;
      GlobalConfig_out.Ki_id=ElectricalID_FOC_output.Ki_id_out;
      GlobalConfig_out.Ki_iq=ElectricalID_FOC_output.Ki_iq_out;
      GlobalConfig_out.Ki_n=ElectricalID_FOC_output.Ki_n_out;
      exit:
    state duringTwoMassID
      entry:
      ControlFlags.startTwoMassID=boolean(0);
      during:
      exit:
    state duringFrictionID
      entry:
      ControlFlags.startFrictionID=boolean(0);
      during:
      exit:
    state duringFluxMapID
      entry:
      ControlFlags.startFluxMapID=boolean(0);
      during:
      exit:
    state finishedFrictionID
      entry:
      finishedFrictionID_loc=uint16(2);
      during:
      exit:
      ControlFlags.transNr=uint16(0);
    state finishedFluxMapID
      entry:
      finishedFluxMapID_loc=uint16(2);
      during:
      exit:
      ControlFlags.transNr=uint16(0);
    state finishedTwoMassID
      entry:
      finishedTwoMassID_loc=uint16(2);
      during:
      exit:
      ControlFlags.transNr=uint16(0);
    state finishedElectricalID
      entry:
      finishedElectricalID_loc=uint16(2);
      during:
      exit:
      ControlFlags.transNr=uint16(0);
    (default) -> decideMotorID
    decideMotorID -> activateElectricalID [order 1] : [ControlFlags.transNr==1 && finishedElectricalID_loc==0]
    activateElectricalID -> decideMotorID [order 2] : [GlobalConfig_in.ElectricalID==0]
        | {ControlFlags.transNr = 0}
    duringElectricalID -> decideMotorID [order 2] : [GlobalConfig_in.ElectricalID==0]
        | {ControlFlags.transNr = 0}
    finishedElectricalID -> decideMotorID
    finishedTwoMassID -> decideMotorID
    decideMotorID -> activateTwoMassID [order 3] : [ControlFlags.transNr==2 && finishedTwoMassID_loc==0]
    activateTwoMassID -> decideMotorID [order 2] : [GlobalConfig_in.TwoMassID==0]
        | {ControlFlags.transNr = 0}
    duringTwoMassID -> decideMotorID [order 2] : [GlobalConfig_in.TwoMassID==0]
        | {ControlFlags.transNr = 0}
    finishedFrictionID -> decideMotorID
    decideMotorID -> activateFrictionID [order 4] : [ControlFlags.transNr==3 && finishedFrictionID_loc==0]
    activateFrictionID -> decideMotorID [order 2] : [GlobalConfig_in.FrictionID==0]
        | {ControlFlags.transNr = 0}
    duringFrictionID -> decideMotorID [order 2] : [GlobalConfig_in.FrictionID==0]
        | {ControlFlags.transNr = 0}
    finishedFluxMapID -> decideMotorID
    decideMotorID -> activateFluxMapID [order 2] : [ControlFlags.transNr==4 && finishedFluxMapID_loc==0]
    activateFluxMapID -> decideMotorID [order 2] : [GlobalConfig_in.FluxMapID==0]
        | {ControlFlags.transNr = 0}
    duringFluxMapID -> decideMotorID [order 2] : [GlobalConfig_in.FluxMapID==0]
        | {ControlFlags.transNr = 0}
    activateElectricalID -> duringElectricalID [order 1] : [enteredElectricalID==1]
    activateTwoMassID -> duringTwoMassID [order 1] : [enteredTwoMassID==1]
    activateFrictionID -> duringFrictionID [order 1] : [enteredFrictionID==1]
    activateFluxMapID -> duringFluxMapID [order 1] : [enteredFluxMapID==1]
    duringTwoMassID -> finishedTwoMassID [order 1] : [finishedTwoMassID==1]
    duringFrictionID -> finishedFrictionID [order 1] : [finishedFrictionID==1]
    duringFluxMapID -> finishedFluxMapID [order 1] : [finishedFluxMapID==1]
    duringElectricalID -> finishedElectricalID [order 1] : [finishedElectricalID==1]
  state Waiting
    entry:
    initParams;
    %wait for activation of
    %FrictionID
    %donothing
  note: ---
  Waiting -> ControlState [order 1] : [GlobalConfig_in.enableParameterID==1 && ....
      | GlobalConfig_in.Reset==0]
  (default) -> Waiting
  ControlState -> Waiting : [GlobalConfig_in.Reset==1 ||....
      |  GlobalConfig_in.enableParameterID==0]
  Waiting -> Waiting [order 2] : [GlobalConfig_in.Reset==1]
  data: finishedFrictionID input boolean; finishedElectricalID input boolean; finishedTwoMassID input boolean; finishedFluxMapID input boolean; enteredFrictionID input boolean; enteredFluxMapID input boolean; enteredTwoMassID input boolean; enteredElectricalID input boolean; ElectricalID_output input Bus: uz_ParaID_ElectricalID_output_t; finishedElectricalID_loc local; finishedFrictionID_loc local; finishedTwoMassID_loc local; finishedFluxMapID_loc local; ElectricalID_FOC_output input Bus: uz_ParaID_Controller_Parameters_output_t; GlobalConfig_in input Bus: uz_ParaID_GlobalConfig_t; GlobalConfig_out output Bus: uz_ParaID_GlobalConfig_t; ControlFlags output Bus: uz_ParaID_ControlFlags_t; enteredOnlineID input
  function decideIDstates:
    | function decideIDstates
    | %If the specific Identification Part is not selected (==0), treat it, as if
    | %it has finished
    | if(GlobalConfig_in.ElectricalID==0)
    |     finishedElectricalID_loc=uint16(1);
    | elseif(finishedElectricalID==1)
    |     finishedElectricalID_loc=uint16(2);
    | end
    | 
    | if(GlobalConfig_in.FrictionID==0)
    |     finishedFrictionID_loc=uint16(1);
    | elseif(finishedFrictionID==1)
    |      finishedFrictionID_loc=uint16(2);
    | end
    | 
    | if(GlobalConfig_in.TwoMassID==0)
    |     finishedTwoMassID_loc=uint16(1);
    | elseif(finishedTwoMassID==1)
    |     finishedTwoMassID_loc=uint16(2);
    | end
    | 
    | if(GlobalConfig_in.FluxMapID==0)
    |     finishedFluxMapID_loc=uint16(1);
    | elseif(finishedFluxMapID==1)
    |     finishedFluxMapID_loc=uint16(2);    
    | end
    | 
    | if(ControlFlags.finished_all_Offline_states == 0)
    |     %Determine path through the ElectricalID-Stateflows
    |     if(GlobalConfig_in.ElectricalID==1 && enteredElectricalID==0 && finishedElectricalID_loc~=2 && finishedElectricalID==0)
    |             ControlFlags.transNr=uint16(1);
    |             finishedElectricalID_loc = uint16(0);
    |     end
    | 
    |     %Determine path through the TwoMassID-Stateflows
    |     if(GlobalConfig_in.TwoMassID==1 && enteredTwoMassID==0 && finishedElectricalID_loc~=0 && finishedTwoMassID_loc~=2 && finishedTwoMassID==0)
    |             ControlFlags.transNr=uint16(2);
    |             finishedTwoMassID_loc = uint16(0);
    |     end
    |     
    |     %Determine path through the FrictionID-Stateflows
    |     if(GlobalConfig_in.FrictionID==1 && enteredFrictionID==0 && finishedElectricalID_loc~=0....
    |        && finishedTwoMassID_loc~=0 && finishedFrictionID_loc~=2 && finishedFrictionID==0)
    |            ControlFlags.transNr=uint16(3);
    |            finishedFrictionID_loc = uint16(0);
    |     end
    | 
    |     %Determine path through the FluxMapID-Stateflows
    |     if(GlobalConfig_in.FluxMapID==1 && enteredFluxMapID==0 && finishedElectricalID_loc~=0....
    |       && finishedTwoMassID_loc~=0 && finishedFrictionID_loc~=0 && finishedFluxMapID_loc~=2 && finishedFluxMapID==0)
    |             ControlFlags.transNr=uint16(4);
    |             finishedFluxMapID_loc = uint16(0);
    |     end
    | end
    | 
    | if(finishedElectricalID_loc~=0 && finishedTwoMassID_loc~=0 && ....
    |         finishedFrictionID_loc~=0 && finishedFluxMapID_loc~=0)
    |     ControlFlags.finished_all_Offline_states = boolean(1);
    | end
    | 
    | end
  function initParams:
    | function initParams
    | %Initialize Variables
    | finishedElectricalID_loc=uint16(0);
    | finishedFrictionID_loc=uint16(0);
    | finishedTwoMassID_loc=uint16(0);
    | finishedFluxMapID_loc=uint16(0);
    | 
    | %Initialize Outputs
    | ControlFlags.startFrictionID             = boolean(0);
    | ControlFlags.startElectricalID           = boolean(0);
    | ControlFlags.startTwoMassID              = boolean(0);
    | ControlFlags.startFluxMapID              = boolean(0);
    | GlobalConfig_out                         = GlobalConfig_in;
    | ControlFlags.enableOnlineID              = boolean(0);
    | ControlFlags.transNr                     = uint16(0);
    | ControlFlags.finished_all_Offline_states = boolean(0);
    | end

== matlab function uz_ParameterID6ph/InterpMeshGrid ==
  data: FluxMapData output Bus: uz_ParaID_FluxMapsData_t; psi_array_in input; i_rat input; OnlineID_input input
function FluxMapData = fcn(psi_array_in,i_rat,OnlineID_input)
%Author Philipp Gebhardt
% Oktober 2019

%This function is calculating the regular flux maps out of the irregular scatter data array stored in psi_array_in. The Outputs rangeX are containg the flux maps axis information which range is related to 3 times i_rat input.
%Furthermore the temperature dependency of the permanent flux is calculated if there are enough measuring values stored in the delta_psi_array. The temperature constant as well as the estimated error of permanent flux
%at reference temperature are given out on psi_temp_const and psi_temp_error outputs.  Using this temperature dependency the flux maps are updated with the permanent flux offset caused by the temperature which is given
%in on OnlineID_input.Wtemp input. 

%-----------------------------------------------------------------------------------------------------------------------------------------
%initalising Outputs
%-----------------------------------------------------------------------------------------------------------------------------------------

psi_array=zeros(6,100);
psi_array=psi_array_in;
delta_psi=zeros(100,1);

FluxMapData.psid_grid=single(zeros(20,20));
FluxMapData.psiq_grid=single(zeros(20,20));
FluxMapData.id_grid=single(zeros(20,20));
FluxMapData.iq_grid=single(zeros(20,20));
FluxMapData.range_id_Y=single(zeros(1,20));
FluxMapData.range_psid_Y=single(zeros(1,20));
FluxMapData.range_psiq_Y=single(zeros(1,20));
FluxMapData.range_psid_X=single(zeros(1,20));
FluxMapData.range_psiq_X=single(zeros(1,20));
FluxMapData.range_iq_Y=single(zeros(1,20));
FluxMapData.range_iq_X=single(zeros(1,20));
FluxMapData.range_id_X=single(zeros(1,20));
FluxMapData.psi_temp_const=single(0.000001);
FluxMapData.psi_temp_error=single(0);



range_psid_X_in=single(zeros(1,20));
range_psid_Y_in=single(zeros(1,20));
range_psiq_X_in=single(zeros(1,20));
range_psiq_Y_in=single(zeros(1,20));
range_id_X_in=single(zeros(1,20));
range_id_Y_in=single(zeros(1,20));
range_iq_X_in=single(zeros(1,20));
range_iq_Y_in=single(zeros(1,20));


%initalise range of flux maps axis
for t=single(0):single(19)
   range_psid_X_in(t+1)=-3*i_rat+t*4*i_rat/19;
   range_psid_Y_in(t+1)=-3*i_rat+t*6*i_rat/19;
   range_psiq_X_in(t+1)=-3*i_rat+t*4*i_rat/19;
   range_psiq_Y_in(t+1)=-3*i_rat+t*6*i_rat/19;
end

%Calculate flux deviation from amout of measuring values and counter sum,
%to average a big amount of measuring values 

for t=single(1):single(100)
    if (OnlineID_input.delta_psi(t,2)>5)
    delta_psi(t,1)=OnlineID_input.delta_psi(t,1)/OnlineID_input.delta_psi(t,2);
    end
end

%Calculate temperature constant with a regressionline, set second input "1"
%to resist outliers greater than 30% (relative to their neighbours)

[psi_temp_const_test,FluxMapData.psi_temp_error]=regressionline(delta_psi,1);

%check plausibility
if(psi_temp_const_test>0&&FluxMapData.psi_temp_const<10)%in mVs/°C
FluxMapData.psi_temp_const=psi_temp_const_test;
end


%correct temperature offset
 for k=single(1):single(100)
   if(psi_array(3,k)~=0)
    psi_array(5,k)=psi_array(5,k)+(psi_array(4,k)-OnlineID_input.Wtemp)*FluxMapData.psi_temp_const;
    psi_array(4,k)=OnlineID_input.Wtemp;
   end
end





%Inter- and extrapolation of the flux maps 
[FluxMapData.range_psid_X,FluxMapData.range_psid_Y,FluxMapData.psid_grid] = interpol_flux_scatter_psid ([psi_array(1,:);psi_array(2,:);psi_array(5,:);zeros(length(psi_array(1,:)))],range_psid_X_in,range_psid_Y_in);
[FluxMapData.range_psiq_X,FluxMapData.range_psiq_Y,FluxMapData.psiq_grid] = interpol_flux_scatter_psiq ([psi_array(1,:);psi_array(2,:);psi_array(6,:);zeros(length(psi_array(1,:)))],range_psiq_X_in,range_psiq_Y_in);

%initialise range of inverse flux maps axis
for t=single(0):single(19)
   range_id_X_in(t+1)=min(min(FluxMapData.psid_grid))+t*(max(max(FluxMapData.psid_grid))-min(min(FluxMapData.psid_grid)))/19;
   range_id_Y_in(t+1)=min(min(FluxMapData.psiq_grid))+t*(max(max(FluxMapData.psiq_grid))-min(min(FluxMapData.psiq_grid)))/19;
   range_iq_X_in(t+1)=min(min(FluxMapData.psid_grid))+t*(max(max(FluxMapData.psid_grid))-min(min(FluxMapData.psid_grid)))/19;
   range_iq_Y_in(t+1)=min(min(FluxMapData.psiq_grid))+t*(max(max(FluxMapData.psiq_grid))-min(min(FluxMapData.psiq_grid)))/19;
end

%Inter and extrapolate inverse flux maps
[FluxMapData.range_id_X,FluxMapData.range_id_Y,FluxMapData.id_grid] = interpol_flux_scatter_psid ([psi_array(5,:);psi_array(6,:);psi_array(1,:);zeros(length(psi_array(1,:)))],range_id_X_in,range_id_Y_in);
[FluxMapData.range_iq_X,FluxMapData.range_iq_Y,FluxMapData.iq_grid] = interpol_flux_scatter_psiq ([psi_array(5,:);psi_array(6,:);psi_array(2,:);zeros(length(psi_array(1,:)))],range_iq_X_in,range_iq_Y_in);

end

== stateflow chart uz_ParameterID6ph/AutoRefCurrents ==
  settings: updateMethod=DISCRETE  sampleTime=1/d_f_states
  note: Philipp Gebhardt, October2019:
      |
      | Description of Control Reference Stateflow:
      |
      | This Stateflow chart is used to generate an cyclic current reference input of d- and q- current. The combinations are circularly arranged in the radius of imax_in.
      | The inputs niq and nid are the amount of measuring values in q- and d-current axis. The input speed_in is used to automatically control the sign of q-current to avoid
      | regenerative current feedback into the inverter.
  state waitState
    entry:
    %do nothing
    %wait for start
  state superstate
    entry:
    counter=single(19998);
    %counter=single(17498);
    iqcount=single(0);
    idcount=single(-AutoRefCurrentsConfig.id_points/3);
    AutoRefCurrents_output.i_dq_ref.d=single(0);
    AutoRefCurrents_output.i_dq_ref.q=single(0);
    imax=single(0);
    state stepstate
      entry:
      if(ActualValues.omega_m>0)
      imax=abs(AutoRefCurrentsConfig.max_current);
      end
      if(ActualValues.omega_m<0)
      imax=abs(AutoRefCurrentsConfig.max_current)*-1;
      end
      if((AutoRefCurrents_output.i_dq_ref.d*AutoRefCurrents_output.i_dq_ref.d+(imax*iqcount/AutoRefCurrentsConfig.iq_points)^2)^0.5<abs(imax))
      AutoRefCurrents_output.i_dq_ref.q=imax*iqcount/AutoRefCurrentsConfig.iq_points;
      else
      iqcount=single(1);
      AutoRefCurrents_output.i_dq_ref.q=imax*iqcount/AutoRefCurrentsConfig.iq_points;
      end
      if((AutoRefCurrents_output.i_dq_ref.q*AutoRefCurrents_output.i_dq_ref.q+(imax*idcount/AutoRefCurrentsConfig.id_points)^2)^0.5<abs(imax))
      AutoRefCurrents_output.i_dq_ref.d=-1*abs(imax)*idcount/AutoRefCurrentsConfig.id_points;
      else
      idcount=single(-AutoRefCurrentsConfig.id_points/3);
      AutoRefCurrents_output.i_dq_ref.d=-1*abs(imax)*idcount/AutoRefCurrentsConfig.id_points;
      end
      counter=single(0);
    state countstate
      entry:
      if(iqcount<AutoRefCurrentsConfig.iq_points)
      iqcount=iqcount+1;
      else
      iqcount=single(0);
      end
      if(idcount<AutoRefCurrentsConfig.id_points)
      idcount=idcount+1;
      else
      idcount=single(-AutoRefCurrentsConfig.id_points/3);
      end
      during:
      counter=counter+1;
    (default) -> countstate
    countstate -> stepstate : [counter==(2.0/GlobalConfig.sampleTimeISR)]
    stepstate -> countstate : [counter==0]
  (default) -> waitState
  waitState -> superstate : [AutoRefCurrentsConfig.enableCRS==1 &&....
      | AutoRefCurrentsConfig.Reset==0 &&....
      |  GlobalConfig.Reset==0 && GlobalConfig.ACCEPT==1&& ....
      | ControlFlags.finished_all_Offline_states==1]
  superstate -> waitState : [AutoRefCurrentsConfig.enableCRS==0 ||....
      |  AutoRefCurrentsConfig.Reset == 1 ||....
      | GlobalConfig.Reset==1]
      | {AutoRefCurrents_output.i_dq_ref.d=single(0);
      | AutoRefCurrents_output.i_dq_ref.q=single(0)}
  data: iqcount local; idcount local; counter local; ActualValues input Bus: uz_ParaID_ActualValues_t; imax local; GlobalConfig input Bus: uz_ParaID_GlobalConfig_t; AutoRefCurrentsConfig input Bus: uz_ParaID_AutoRefCurrentsConfig_t; AutoRefCurrents_output output Bus: uz_ParaID_AutoRefCurrents_output_t; ControlFlags input Bus: uz_ParaID_ControlFlags_t

== stateflow chart uz_ParameterID6ph/FOC_ControlState ==
  settings: updateMethod=DISCRETE  sampleTime=1/d_f_states
  note: Control-States
  state FOC_ControlState
    entry:
    FOCControl_output.activeState = uint16(600);
    initParams;
    during:
    note: FOC current control
    state FOCcurrentControl 	%state 140
      entry:
      FOCControl_output.activeState = uint16(610);
      FOCControl_output.enableFOC_current=boolean(1);
      counter = uint32(1);
      during:
      FOCControl_output.i_dq_ref.q=GlobalConfig.i_dq_ref.q;
      FOCControl_output.i_dq_ref.d=GlobalConfig.i_dq_ref.d+i_d_Online_ref;
      exit:
      counter = uint32(1);
      FOCControl_output.enableFOC_current=boolean(0);
    state FOCdecider
      entry:
    note: FOC speed control
    note: change speed with sinusoidal trajectory in 0.2 sec
    state FOCspeed_speedChange 	%state 13.0
      entry:
      FOCControl_output.activeState = uint16(620);
      FOCControl_output.enableFOC_speed=boolean(1);
      counter = uint32(1);
      during:
      FOCControl_output.i_dq_ref.d = i_d_Online_ref+GlobalConfig.i_dq_ref.d;
      n_filt = single((single(counter)*GlobalConfig.sampleTimeISR*5)-....
      1/(2*pi)*sin(2*pi*single(counter)*GlobalConfig.sampleTimeISR*5));
      FOCControl_output.n_ref_FOC=((GlobalConfig.n_ref-n_ref_old)*n_filt)+n_ref_old;
      counter = counter + 1;
      exit:
      counter = uint32(1);
    state FOCspeed_constantSpeed 		%state 13.1
      entry:
      FOCControl_output.activeState = uint16(621);
      n_ref_old = GlobalConfig.n_ref;
      during:
      FOCControl_output.n_ref_FOC=GlobalConfig.n_ref;
      FOCControl_output.i_dq_ref.d=GlobalConfig.i_dq_ref.d +i_d_Online_ref;
      exit:
      counter = uint32(1);
      FOCControl_output.enableFOC_speed=boolean(0);
      note: constant speed
    (default) -> FOCdecider
    FOCdecider -> FOCcurrentControl 	%state 140 [order 1] : [controlType==0]
    FOCdecider -> FOCspeed_speedChange 	%state 13.0 [order 2] : [controlType==1]
    FOCspeed_constantSpeed 		%state 13.1 -> FOCspeed_speedChange 	%state 13.0 : [GlobalConfig.n_ref~=n_ref_old]
    FOCspeed_speedChange 	%state 13.0 -> FOCspeed_constantSpeed 		%state 13.1 : after(0.2,sec)
  state Waiting
    entry:
    %wait for activation of
    %FOCcontrol
    %donothing
  note: ---
  Waiting -> FOC_ControlState : [GlobalConfig.Reset==0 && ControlFlags.finished_all_Offline_states==1]
  (default) -> Waiting
  FOC_ControlState -> Waiting : [GlobalConfig.Reset==1]
  data: n_ref_old local; n_filt local; i_d_R_online local; counter local; FOCControl_output output Bus: uz_ParaID_Controller_Parameters_output_t; J local; measArray1 local; d local; i_d_Online_ref input; GlobalConfig input Bus: uz_ParaID_GlobalConfig_t; ControlFlags input Bus: uz_ParaID_ControlFlags_t; controlType input
  function initParams:
    | function initParams
    | 
    | % initialize variables
    | n_filt              = single(0.0);
    | n_ref_old           = single(0.0);
    | counter 			= uint32(1);
    | measArray1			= single(zeros(1024,1));
    | i_d_R_online        = single(0.0);
    | d        			= single(zeros(2048,1));
    | J 					= single(zeros(2048,2));
    | 
    | %Outputs
    | FOCControl_output.Ki_n_out          = single(GlobalConfig.Ki_n);
    | FOCControl_output.Ki_iq_out         = single(GlobalConfig.Ki_iq);
    | FOCControl_output.Ki_id_out         = single(GlobalConfig.Ki_id);
    | FOCControl_output.Kp_n_out          = single(GlobalConfig.Kp_n);
    | FOCControl_output.Kp_iq_out         = single(GlobalConfig.Kp_iq);
    | FOCControl_output.Kp_id_out         = single(GlobalConfig.Kp_id);
    | FOCControl_output.n_ref_FOC         = single(0.0);
    | FOCControl_output.i_dq_ref.d        = single(0.0);
    | FOCControl_output.i_dq_ref.q        = single(0.0);
    | FOCControl_output.i_dq_ref.zero      = single(0.0);
    | FOCControl_output.enableFOC_speed   = boolean(0);
    | FOCControl_output.enableFOC_current	= boolean(0);
    | FOCControl_output.resetIntegrator   = boolean(0);
    | FOCControl_output.activeState       = uint16(0);
    | 
    | end
